simulink model "TrafficLightDemo"  (R2023a)
settings: Solver=VariableStepAuto  StartTime=0.0  StopTime=Inf  RelTol=1e-3
settings Model: Creator=splas  LastModifiedBy=splas

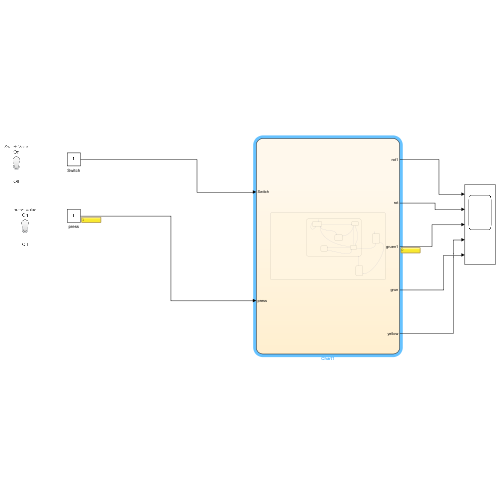
[thumbnail: Simulink's stored preview of the top-level diagram]
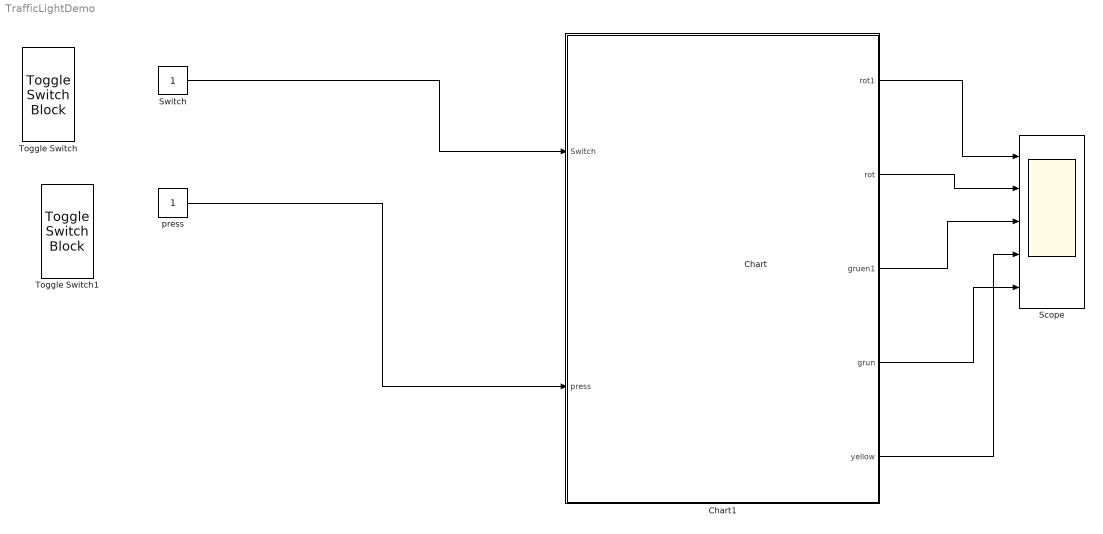
== system TrafficLightDemo ==
  Chart : Stateflow chart  TreatAsAtomicUnit=on
  Chart1 : Stateflow chart  TreatAsAtomicUnit=on
      settings: PortSchema="{\"entries\":[{\"content\":{\"sides\":[{\"content\":{\"connectorIds\":[\"In2\",\"In1\"]},\"type\":\"ConnectorPlacement.EquallySpacedRectSide\",\"uuid\":\"4fda1b98-2af6-4351-880e-f9bdc70e47dd\"},{\"content\":{\"connectorIds\":[\"Out1\",\"Out2\",\"Out3\",\"Out5\",\"Out4\"],\"side\":\"RIGHT\"},\"type\":\"ConnectorPlacement.EquallySpacedRectSide\",\"uuid\":\"94420cfc-6b2b-438e-8ee2-c97ac7c28afd\"},{\"content\":{\"side\":\"TOP\"},\"type\":\"ConnectorPlacement.EquallySpacedRectSide\",\"uuid\":\"e19f0192-5f31-43c3-93c5-98f3d346d4de\"}]},\"type\":\"ConnectorPlacement.EquallySpacedConnector\",\"uuid\":\"f20e8edb-3a85-432a-a054-5846a1c25842\"}],\"packageUris\":[\"http://schema.mathworks.com/mf0/Connector/R2020b\"],\"version\":\"1.0\"}"
  Scope : Scope  NumInputPorts=5
  Switch : Constant
  Toggle Switch : ToggleSwitchBlock
      settings: Values={{'Off', 'On'}, [0 1]}
  Toggle Switch1 : ToggleSwitchBlock
      settings: Values={{'Off', 'On'}, [0 1]}
  press : Constant
  wires:
  press/1 -> Chart1/1(press)
  Chart1/1(rot1) -> Scope/1
  Chart1/2(rot) -> Scope/2
  Chart1/3(gruen1) -> Scope/3
  Chart1/4(yellow) -> Scope/4
  Chart1/5(grun) -> Scope/5
  Switch/1 -> Chart1/2(Switch)

== stateflow chart TrafficLightDemo/Chart1 ==
  state Traffic
    en: x= 0;
    state Light_Change
      state GelbS
        en:yellow = 1;
        ex:yellow=0;
      state GelbS_RotF
        en:rot1 = 1;
        en:yellow=1;
      state GrunS_RotF
        en:grun=1;
        en:rot1=1;
        en:yellow=0;
        en:rot=0;
        ex:grun= 0;
      state RotS_RotF
        en:rot=1;
        en:rot1 = 1;
        en:yellow = 0;
      state RotS_Gr_nF
        en:gruen1 = 1;
        en:rot= 1;
        en:rot1= 0;
        ex:gruen1 = 0;
      (default) -> GelbS
      GelbS -> GelbS [order 3] : [after(1,sec)&&x == 0]{x= x+1}
      GelbS -> GelbS_RotF [order 1] : after(3,sec)[x == 1]{x = x+1}
      GrunS_RotF -> GelbS_RotF : [(press == 1&&x ==7&&after(20,sec)) || after(40,sec)]{x = x+1}
      GelbS_RotF -> RotS_RotF [order 1] : after(10,sec)[x ==2]{x = x+1}
      GelbS_RotF -> RotS_RotF [order 2] : [after(2,sec)&&x ==8]{x = x+1}
      RotS_RotF -> GelbS [order 3] : after(2,sec)[x == 5]{x = x+1}
      GelbS -> GrunS_RotF [order 2] : after(2,sec)[x == 6]{x=x+1}
      RotS_RotF -> RotS_Gr_nF [order 1] : after(5,sec)[x == 3]{x = x+1}
      RotS_Gr_nF -> RotS_RotF : after(15,sec)[x == 4]{x=x+1}
    state Aus
      en:yellow = 0;
      en:rot1 = 0;
      en:rot = 0;
      en:grun= 0;
      en:gruen1 = 0;
    state An
      en:yellow = 1;
      en:rot1 = 0;
      en:rot = 0;
      en:grun= 0;
      en:gruen1 = 0;
      en:x = 0;
    (default) -> Aus
    Aus -> An : [Switch == 1]
    RotS_RotF -> Aus [order 2] : [Switch == 0 ||(x ==9&&after(10,sec))]
    An -> Light_Change : [Switch == 1]
  data: press input; Switch input; rot1 output uint8; rot output uint8; gruen1 output uint8; yellow output uint8; grun output uint8; x local

== stateflow chart TrafficLightDemo/Chart ==
